simulink model "rpend"  (R2017a)
settings: Solver=FixedStepDiscrete  StartTime=0.0  StopTime=inf  FixedStep=Ts  RelTol=1e-3  EnableMultiTasking=on
model workspace (MAT data in the model file):
  A = [0.725776748419  0  0  0  0; 0.00140279437205  0.999944490331  -5.55096688988e-05  0.000560056855223  -1.53017606364e-07; -0.00302972158237  0.00580760965337  1.00580760965  0.0204062816553  0.0100132446668; 0.127342671518  -0.00589430256759  -0.00589430256759  -9.08670431161e-05  -4.38663519616e-05; -0.275479681015  1.15113945046  1.15113945046  2.16826031914  1.00457363851]
  B = [-11.2592502197; -0.00918249434523; 0.019826227923; -1.84605491293; 3.98706504917]
  C = [0  1  0  0  0; 0  0  1  0  0]
  D = [0; 0]
  K = [-0.0237640315485 7.87586462007 6.73482643041 1.33377274874 0.619465225229]
  L = [263.012994947  0.303996367845; 1.53081831637  0.000653840106358; 0.603953784827  1.8170329595; 46.1341519736  0.0439034608107; 78.3867491864  83.4953194858]
  L1 = 1
  L2 = 1.1
  Q = [1  0  0  0  0; 0  10000  0  0  0; 0  0  100000  0  0; 0  0  0  100  0; 0  0  0  0  1]
  R = 60000
  Ts = 0.01
  g = 9.81
  h = 0.01
  initial_state = [0 0]
  par.g = 9.81
  par.L1 = 1
  par.L2 = 1.1
  par.k_m = 41.0587
  par.tau_e = 0.0312
values from neighbouring files (symbols this model uses):
  adingain = [adingain 1 1 1 1 1]    [hwinit.m]
  adinoffs = [adinoffs 0 0 0 0 0]    [hwinit.m]
  daoutgain = 1*[-6]    [hwinit.m]
  daoutoffs = [0.00]    [hwinit.m]
undefined symbols (not defined in the file or in its folder): Discrete, Time
libraries: ctrlSharedLib x1
settings Model: Creator=rbabuska  LastModifiedBy=Ortix
settings DataIOCC: LimitDataPoints=on  SaveFormat=Array  SignalLoggingName=sigsOut
settings OptimizationCC: BooleanDataType=off  ExpressionDepthLimit=2147483647  InitFltsAndDblsToZero=on  LifeSpan=inf
settings DebuggingCC: SaveWithParameterizedLinksMsg=none  SignalResolutionControl=TryResolveAllWithWarning  MultiTaskDSMMsg=warning  MultiTaskCondExecSysMsg=none  AllowSymbolicDim=off  StateNameClashWarn=warning  SFUnexpectedBacktrackingDiag=warning  SFNoUnconditionalDefaultTransitionDiag=warning  SFExecutionAtInitializationDiag=none
settings HardwareCC: ProdBitPerPointer=32  ProdBitPerSizeT=32  ProdBitPerPtrDiffT=32  ProdLargestAtomicFloat=None  ProdIntDivRoundTo=Undefined  ProdEndianess=Unspecified  ProdWordSize=32  ProdHWDeviceType=32-bit Generic  TargetUnknown=on
settings ModelReferenceCC: PropagateSignalLabelsOutOfModel=off
settings GRTTargetCC: TargetFcnLib=ansi_tfl_tmw.mat  TargetLangStandard=C89/C90 (ANSI)  GeneratePreprocessorConditionals=Disable all  CombineOutputUpdateFcns=off  GRTInterface=on
settings ConfigComp: CovMetricSettings=dw  CovHtmlReporting=on  CovSaveCumulativeToWorkspaceVar=on  CovSaveSingleToWorkspaceVar=on  CovExternalEMLEnable=off

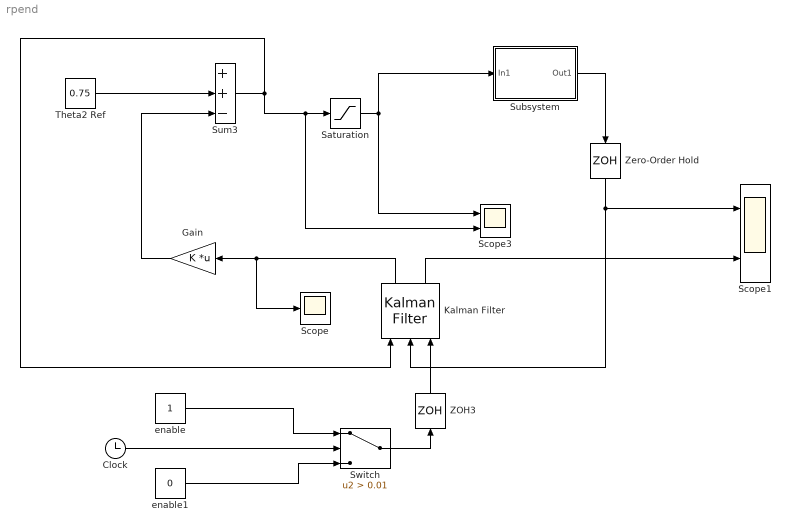
== system rpend ==
  Clock : Clock
  Gain : Gain  Gain=K  Multiplication=Matrix(K*u)
  Kalman Filter : ctrlSharedLib/Kalman Filter  TimeDomain=Discrete-Time  UseCurrentEstimator=on  ModelSource=Individual A, B, C, D matrices  ModelSourceVariable=sys  A=A  B=B  C=C  D=D  NumberOfStates=2  NumberOfInputs=2  NumberOfOutputs=2  InitialEstimateSource=Dialog  X0=[0 0 0 0 0]  P0=10  UseK=off  UseGH=off  NumberOfProcessNoiseInputs=2  G=1  TimeInvariantG=on  H=0  TimeInvariantH=on  Q=Q  TimeInvariantQ=on  R=R  TimeInvariantR=on  N=0  TimeInvariantN=on  AddInputPort=on  AddEnablePort=on  OutputEstimatedY=on  OutputP=off  Ts=Ts
  Saturation : Saturate  UpperLimit=1  LowerLimit=-1
  Scope : Scope
  Scope1 : Scope  NumInputPorts=2
  Scope3 : Scope  NumInputPorts=2
  Subsystem : Subsystem
      mask Display: disp('Rotational\nPendulum')
  Sum3 : Sum  Inputs=++-
  Switch : Switch  Criteria=u2 > Threshold  Threshold=0.01
  Theta2 Ref : Constant  Value=0.75
  ZOH3 : ZeroOrderHold  SampleTime=Ts
  Zero-Order Hold : ZeroOrderHold  SampleTime=Ts
  enable : Constant  SampleTime=Ts
  enable1 : Constant  Value=0  SampleTime=Ts
  wires:
  Theta2 Ref/1 -> Sum3/2
  Sum3/1 -> Kalman Filter/1, Scope3/2, Saturation/1
  Gain/1 -> Sum3/3
  Kalman Filter/2 -> Scope1/2
  Subsystem/1(Out1) -> Zero-Order Hold/1
  Kalman Filter/1 -> Gain/1, Scope/1
  Saturation/1 -> Subsystem/1(In1), Scope3/1
  Zero-Order Hold/1 -> Scope1/1, Kalman Filter/2
  Switch/1 -> ZOH3/1
  Clock/1 -> Switch/2
  enable/1 -> Switch/1
  enable1/1 -> Switch/3
  ZOH3/1 -> Kalman Filter/3

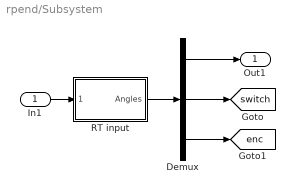
== system rpend/Subsystem ==
  In1 : Inport
  Demux : Demux  Outputs=[2 4 1]
  RT input : Subsystem  mask{Ts=h, channels=[6 7]}
      mask prompts: Ts "Sample time [s]:"; channels "Channels to read (e.g., [6 7])"
      mask init:
      | hwinit;
      | 
      | % initialize FPGA
      | fugihandle = fugiboard('Open', 'Pendulum1');
      | fugihandle.WatchdogTimeout = 0.5;
      | fugiboard('SetParams', fugihandle);
      | fugiboard('Write', fugihandle, 0, 0, 0, 0);  % dummy write to sync interface board
      | fugiboard('Write', fugihandle, 5, 1, 0, 0);  % reset position, activate relay
      | data = fugiboard('Read', fugihandle);        % get version info from FPGA
      | % model = bitshift(data(1), -5); 
      | % version = bitand(data(1), 31);
      | % disp(sprintf('FPGA setup %d, version %d', model, version)); % for the B&P it should say 1 1, or else there is a problem
      | fugiboard('Write', fugihandle, 0, 1, 0, 0);  % end reset
      | pause(0.1);                         % give relay some time to respond
      mask Display: disp('Rotational\nPendulum')
  Out1 : Outport
  tag scope: enc=global, switch=global
  wires:
  RT input/1(Angles) -> Demux/1
  Demux/1 -> Out1/1
  Demux/2 -> [switch]
  Demux/3 -> [enc]
  In1/1 -> RT input/1(Motors)

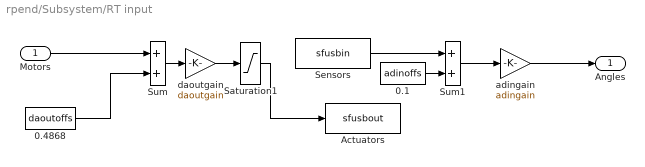
== system rpend/Subsystem/RT input ==
  Motors : Inport
  0.1 : Constant  Value=adinoffs
  0.4868 : Constant  Value=daoutoffs
  Actuators : S-Function  FunctionName=sfusbout  Parameters=Ts, fugihandle  SFunctionDeploymentMode=off  EnableBusSupport=off
  Saturation1 : Saturate  UpperLimit=10  LowerLimit=-10
  Sensors : S-Function  FunctionName=sfusbin  Parameters=Ts, fugihandle, channels  SFunctionDeploymentMode=off  EnableBusSupport=off
  Sum : Sum  SaturateOnIntegerOverflow=on  InputSameDT=on  OutDataTypeStr=Inherit: Same as first input
  Sum1 : Sum  SaturateOnIntegerOverflow=on  InputSameDT=on  OutDataTypeStr=Inherit: Same as first input
  adingain : Gain  Gain=adingain  SaturateOnIntegerOverflow=on  OutDataTypeStr=Inherit: Same as input  ParamDataTypeStr=Inherit: Same as input
  daoutgain : Gain  Gain=daoutgain  SaturateOnIntegerOverflow=on  OutDataTypeStr=Inherit: Same as input  ParamDataTypeStr=Inherit: Same as input
  Angles : Outport
  wires:
  Sum/1 -> daoutgain/1
  0.4868/1 -> Sum/2
  Motors/1 -> Sum/1
  Sum1/1 -> adingain/1
  0.1/1 -> Sum1/2
  Sensors/1 -> Sum1/1
  adingain/1 -> Angles/1
  Saturation1/1 -> Actuators/1
  daoutgain/1 -> Saturation1/1
